simulink model "CANOnlineTest"  (R2020a)
settings: Solver=ode1  StartTime=0.0  StopTime=10  FixedStep=Ts  RelTol=1e-3  EnableMultiTasking=on
undefined symbols (not defined in the file): AMR, Ts
libraries: simulink x2, dspsigops x1, discrete_timer x1
settings Model: Creator=tbria  LastModifiedBy=Harjot
settings OptimizationCC: LifeSpan=inf
settings DebuggingCC: SFUnexpectedBacktrackingDiag=warning  SFNoUnconditionalDefaultTransitionDiag=warning  SFExecutionAtInitializationDiag=none  ArithmeticOperatorsInVariantConditions=warning
settings SFSimCC: SimUseLocalCustomCode=off  CustomCodeUndefinedFunction=UseInterfaceOnly
settings RTWCC: RTWUseLocalCustomCode=off
settings CodeAppCC: StateflowObjectComments=on
settings GRTTargetCC: TargetLangStandard=C89/C90 (ANSI)
settings ConfigComp: CovMetricSettings=dw  CovHtmlReporting=on  CovSaveCumulativeToWorkspaceVar=on  CovSaveSingleToWorkspaceVar=on  CovExternalEMLEnable=off

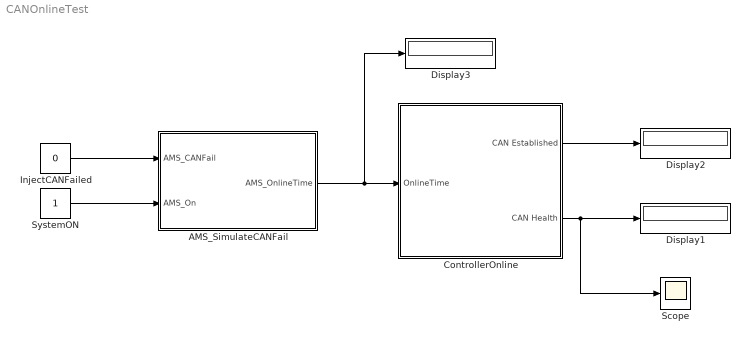
== system CANOnlineTest ==
  AMS_SimulateCANFail : Subsystem
  ControllerOnline : Subsystem
  Display1 : Display
  Display2 : Display
  Display3 : Display
  InjectCANFailed : Constant  Value=0
  Scope : Scope
  SystemON : Constant
  wires:
  InjectCANFailed/1 -> AMS_SimulateCANFail/1(AMS_CANFail)
  AMS_SimulateCANFail/1(AMS_OnlineTime) -> Display3/1, ControllerOnline/1(OnlineTime)
  ControllerOnline/1(CAN Established) -> Display2/1
  ControllerOnline/2(CAN Health) -> Scope/1, Display1/1
  SystemON/1 -> AMS_SimulateCANFail/2(AMS_On)

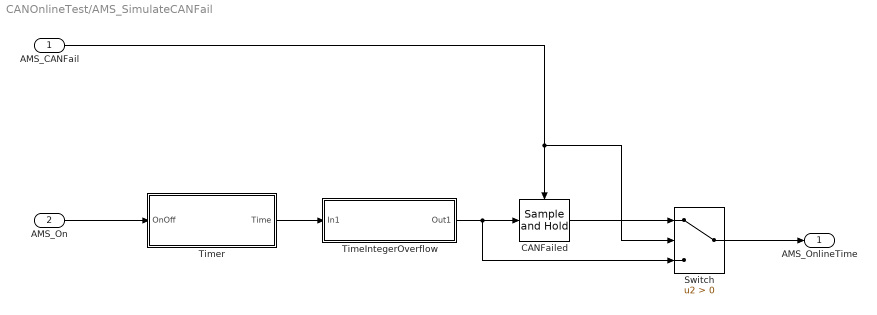
== system CANOnlineTest/AMS_SimulateCANFail ==
  AMS_CANFail : Inport
  AMS_On : Inport  Port=2
  CANFailed : dspsigops/Sample and Hold  trig=Rising edge  initCond=0  latchinput=off
  Switch : Switch  Criteria=u2 > Threshold
  TimeIntegerOverflow : Subsystem
  Timer : Subsystem
  AMS_OnlineTime : Outport  VectorParamsAs1DForOutWhenUnconnected=off
  wires:
  Switch/1 -> AMS_OnlineTime/1
  CANFailed/1 -> Switch/1
  AMS_CANFail/1 -> Switch/2, CANFailed/Trigger
  Timer/1(Time) -> TimeIntegerOverflow/1(In1)
  TimeIntegerOverflow/1(Out1) -> Switch/3, CANFailed/1
  AMS_On/1 -> Timer/1(OnOff)

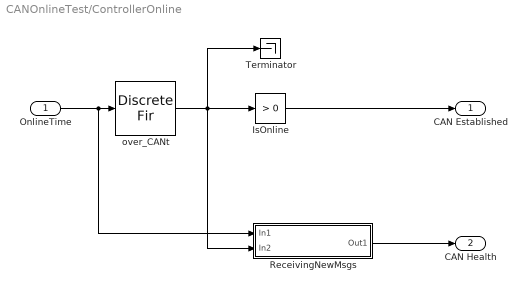
== system CANOnlineTest/ControllerOnline ==
  OnlineTime : Inport
  IsOnline : simulink/Logic and Bit Operations/Compare To Zero  relop=>  OutDataTypeStr=boolean
  ReceivingNewMsgs : Subsystem
  Terminator : Terminator
  over_CANt : DiscreteFir  Coefficients=[ones(1,AMR.CAN.Timeout.t/Ts)./(AMR.CAN.Timeout.t/Ts)]  InputProcessing=Columns as channels (frame based)  SampleTime=Ts
  CAN Established : Outport  VectorParamsAs1DForOutWhenUnconnected=off
  CAN Health : Outport  Port=2  VectorParamsAs1DForOutWhenUnconnected=off
  wires:
  over_CANt/1 -> Terminator/1, ReceivingNewMsgs/2(In2), IsOnline/1
  OnlineTime/1 -> ReceivingNewMsgs/1(In1), over_CANt/1
  IsOnline/1 -> CAN Established/1
  ReceivingNewMsgs/1(Out1) -> CAN Health/1

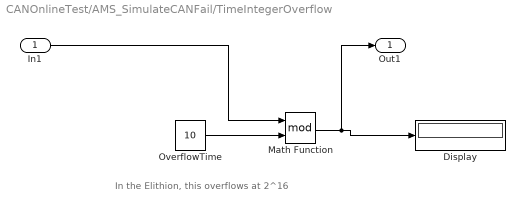
== system CANOnlineTest/AMS_SimulateCANFail/TimeIntegerOverflow ==
  note: In the Elithion, this overflows at 2^16
  In1 : Inport
  Display : Display
  Math Function : Math  Operator=mod  SignedPower=on  SaturateOnIntegerOverflow=on
  OverflowTime : Constant  Value=10
  Out1 : Outport  VectorParamsAs1DForOutWhenUnconnected=off
  wires:
  OverflowTime/1 -> Math Function/2
  In1/1 -> Math Function/1
  Math Function/1 -> Out1/1, Display/1

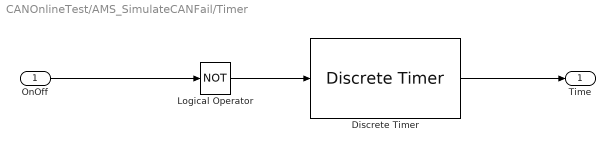
== system CANOnlineTest/AMS_SimulateCANFail/Timer ==
  OnOff : Inport
  Discrete Timer : discrete_timer/Discrete Timer
  Logical Operator : Logic  Operator=NOT  Inputs=1  AllPortsSameDT=off  OutDataTypeStr=boolean
  Time : Outport  VectorParamsAs1DForOutWhenUnconnected=off
  wires:
  Discrete Timer/1 -> Time/1
  Logical Operator/1 -> Discrete Timer/1
  OnOff/1 -> Logical Operator/1

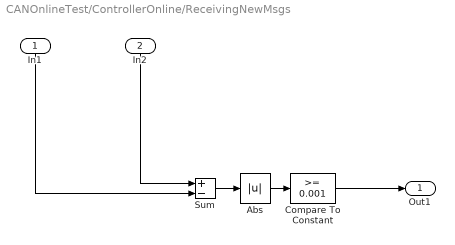
== system CANOnlineTest/ControllerOnline/ReceivingNewMsgs ==
  In1 : Inport
  In2 : Inport  Port=2
  Abs : Abs
  Compare To Constant : simulink/Logic and Bit Operations/Compare To Constant  relop=>=  const=0.001  OutDataTypeStr=boolean
  Sum : Sum  Inputs=+-
  Out1 : Outport  VectorParamsAs1DForOutWhenUnconnected=off
  wires:
  Abs/1 -> Compare To Constant/1
  Compare To Constant/1 -> Out1/1
  Sum/1 -> Abs/1
  In2/1 -> Sum/1
  In1/1 -> Sum/2
